simulink model "w1prob6"  (R2020a)
settings: Solver=VariableStepAuto  StartTime=0.0  StopTime=10.0  RelTol=1e-3
libraries: simulink x1
settings Model: Creator=Anjali123  LastModifiedBy=Anjali123

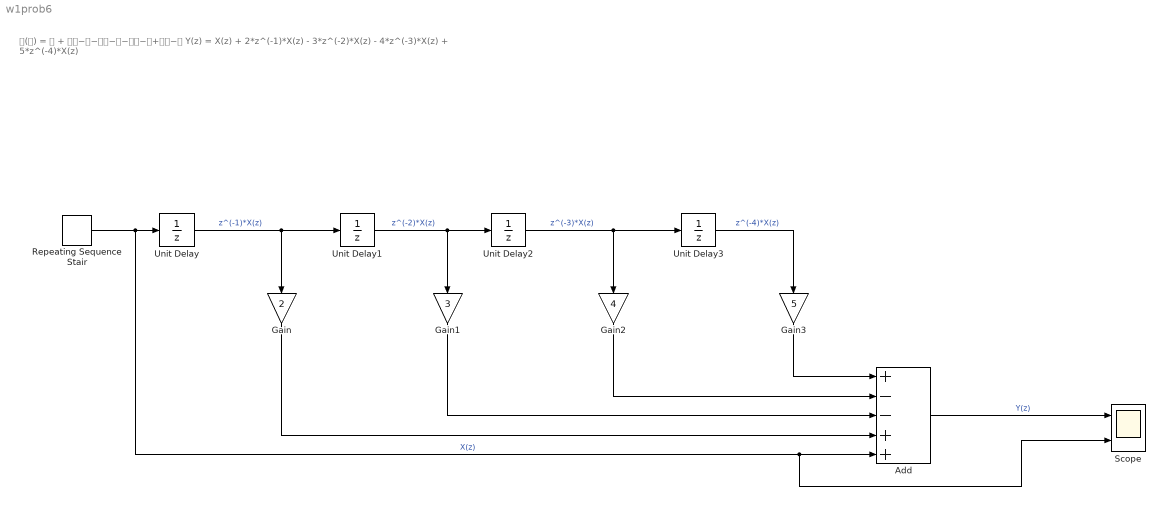
== system w1prob6 ==
  note: 𝐇(𝐳) = 𝟏 + 𝟐𝐳−𝟏−𝟑𝐳−𝟐−𝟒𝐳−𝟑+𝟓𝐳−𝟒
      | Y(z) = X(z) + 2*z^(-1)*X(z) - 3*z^(-2)*X(z) - 4*z^(-3)*X(z) + 5*z^(-4)*X(z)
  Add : Sum  Inputs=+--++
  Gain : Gain  Gain=2
  Gain1 : Gain  Gain=3
  Gain2 : Gain  Gain=4
  Gain3 : Gain  Gain=5
  Repeating Sequence Stair : simulink/Sources/Repeating Sequence Stair  OutValues=[3 1 4 2 1].'  tsamp=-1  OutMin=[]  OutMax=[]  OutDataTypeStr=double  OutputDataTypeScalingMode=double  OutDataType=fixdt(0,8)  ConRadixGroup=Best Precision: Vector-wise  OutScaling=2^-12
  Scope : Scope  NumInputPorts=2
  Unit Delay{,1..3} (4 alike) : UnitDelay  SampleTime=-1  HasFrameUpgradeWarning=on
  wires:
  Repeating Sequence Stair/1 -> Scope/2, Add/5, Unit Delay/1  "X(z)"
  Unit Delay/1 -> Unit Delay1/1, Gain/1  "z^(-1)*X(z)"
  Gain/1 -> Add/4
  Unit Delay1/1 -> Gain1/1, Unit Delay2/1  "z^(-2)*X(z)"
  Unit Delay2/1 -> Gain2/1, Unit Delay3/1  "z^(-3)*X(z)"
  Unit Delay3/1 -> Gain3/1  "z^(-4)*X(z)"
  Gain3/1 -> Add/1
  Gain2/1 -> Add/2
  Gain1/1 -> Add/3
  Add/1 -> Scope/1  "Y(z)"
